simulink model "state_obsv"  (R2020b)
settings: Solver=VariableStepAuto  StartTime=0.0  StopTime=1  MaxStep=1e-3  RelTol=1e-3
values from neighbouring files (symbols this model uses):
  A = [-R/L -1/L; 1/Ca 0]    [E1_1.m]    (also in E3_5.m = [-299 37;-2416 299]; E5_1.m = [0 0 1; 2 -1 2; 0 1 1]; E_140421_1.m = [0 -1; 3 -2]; E_140421_2.m = [3 2; 0 -5])
  alpha = 1    [Reg.m]    (also in State_feed.m = [-(C-D*K)*(A-B*K)^-1*B+D]^-1)
  B = [1/L 0]'    [E1_1.m]    (also in E3_5.m = [7 57]'; E_140421_1.m = [1 1]'; E_140421_2.m = [1 0]'; E_280421_1.m = [1;2])
  C = [0 1]    [E1_1.m]    (also in E5_1.m = [0 0 1]; E_140421_1.m = [1 1]; E_140421_2.m = [1 1]; E_280421_1.m = [1 -1])
  K = place(A,B,[-1 -7])    [E3_5.m]    (also in E_140421_1.m = place(A,B,[20 -10]); Esempi.m = place(A,B,[-1,-2,-3]); EserciziFinali.m = place(A,B,[20, -10]); Problem_P2.m = 20*log10(m))
  L = 2e-3    (= 0.002)    [E1_1.m]    (also in E5_1.m = Lt'; Esempi.m = place(A',C',[0.05 0.1 0.2])'; EserciziFinali.m = place(A',C',[-10 -20])'; Exam_202007.m = Gc*Gp*Gs*Ga*Gf)
libraries: simulink x1
settings Model: Creator=kevin  LastModifiedBy=kevin

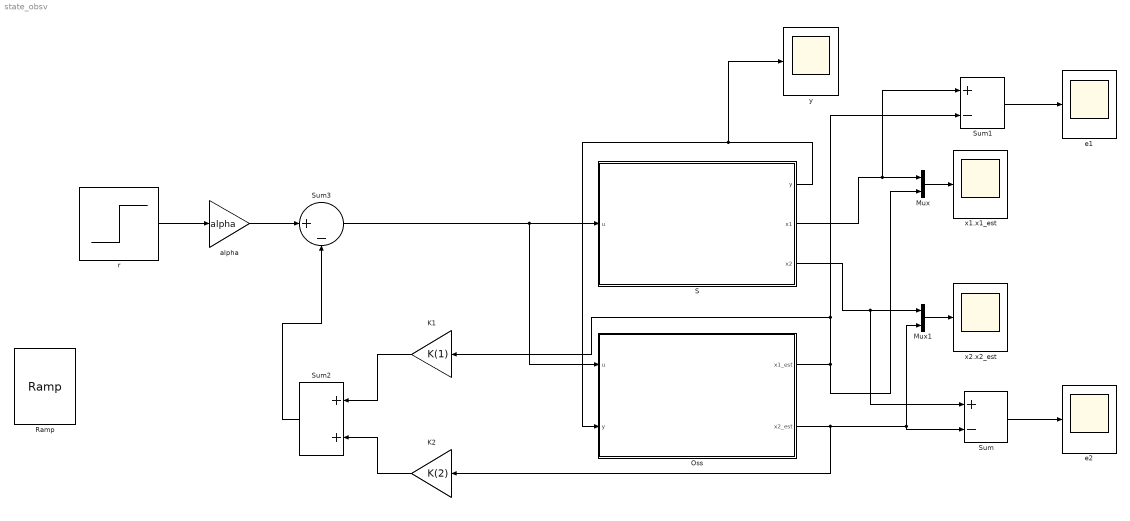
== system state_obsv ==
  K1 : Gain  Gain=K(1)
  K2 : Gain  Gain=K(2)
  Mux : Mux  Inputs=2
  Mux1 : Mux  Inputs=2
  Oss : Subsystem
  Ramp : simulink/Sources/Ramp  slope=1  start=0  InitialOutput=0
  S : Subsystem
  Sum : Sum  Inputs=+-
  Sum1 : Sum  Inputs=+-
  Sum2 : Sum
  Sum3 : Sum  Inputs=|+-
  alpha : Gain  Gain=alpha
  e1 : Scope
  e2 : Scope
  r : Step  Time=0  SampleTime=0
  x1.x1_est : Scope
  x2.x2_est : Scope
  y : Scope
  wires:
  Mux/1 -> x1.x1_est/1
  Mux1/1 -> x2.x2_est/1
  S/2(x1) -> Sum1/1, Mux/1
  S/3(x2) -> Sum/1, Mux1/1
  Oss/2(x2_est) -> K2/1, Sum/2, Mux1/2
  S/1(y) -> y/1, Oss/2(y)
  Sum1/1 -> e1/1
  Sum/1 -> e2/1
  Oss/1(x1_est) -> Mux/2, K1/1, Sum1/2
  r/1 -> alpha/1
  alpha/1 -> Sum3/1
  Sum2/1 -> Sum3/2
  K2/1 -> Sum2/2
  K1/1 -> Sum2/1
  Sum3/1 -> Oss/1(u), S/1(u)

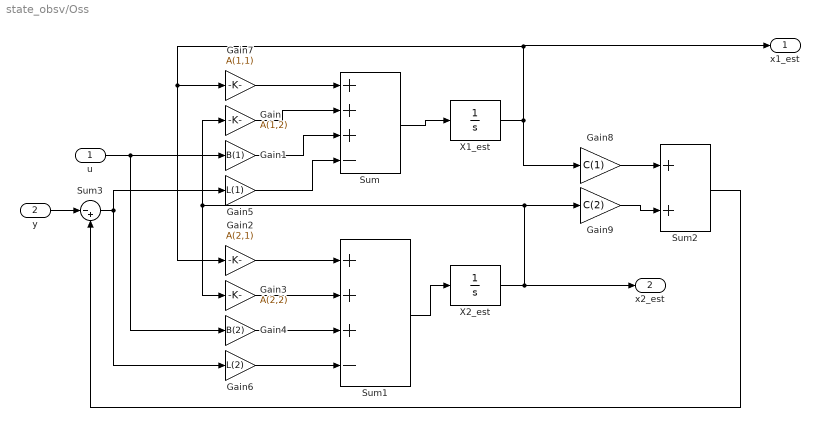
== system state_obsv/Oss ==
  u : Inport
  y : Inport  Port=2
  Gain : Gain  Gain=A(1,2)
  Gain1 : Gain  Gain=B(1)
  Gain2 : Gain  Gain=A(2,1)
  Gain3 : Gain  Gain=A(2,2)
  Gain4 : Gain  Gain=B(2)
  Gain5 : Gain  Gain=L(1)
  Gain6 : Gain  Gain=L(2)
  Gain7 : Gain  Gain=A(1,1)
  Gain8 : Gain  Gain=C(1)
  Gain9 : Gain  Gain=C(2)
  Sum : Sum  Inputs=+++-
  Sum1 : Sum  Inputs=+++-
  Sum2 : Sum
  Sum3 : Sum  Inputs=|-+
  X1_est : Integrator
  X2_est : Integrator
  x1_est : Outport
  x2_est : Outport  Port=2
  wires:
  Gain4/1 -> Sum1/3
  Sum/1 -> X1_est/1
  X2_est/1 -> x2_est/1, Gain9/1, Gain3/1, Gain/1
  Gain3/1 -> Sum1/2
  Sum1/1 -> X2_est/1
  Gain/1 -> Sum/2
  Gain1/1 -> Sum/3
  u/1 -> Gain4/1, Gain1/1
  X1_est/1 -> Gain8/1, Gain7/1, Gain2/1, x1_est/1
  Gain2/1 -> Sum1/1
  Sum2/1 -> Sum3/2
  y/1 -> Sum3/1
  Sum3/1 -> Gain6/1, Gain5/1
  Gain5/1 -> Sum/4
  Gain6/1 -> Sum1/4
  Gain7/1 -> Sum/1
  Gain8/1 -> Sum2/1
  Gain9/1 -> Sum2/2

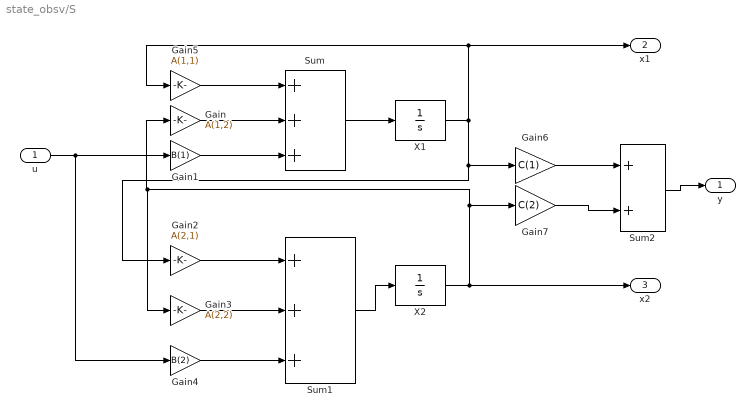
== system state_obsv/S ==
  u : Inport
  Gain : Gain  Gain=A(1,2)
  Gain1 : Gain  Gain=B(1)
  Gain2 : Gain  Gain=A(2,1)
  Gain3 : Gain  Gain=A(2,2)
  Gain4 : Gain  Gain=B(2)
  Gain5 : Gain  Gain=A(1,1)
  Gain6 : Gain  Gain=C(1)
  Gain7 : Gain  Gain=C(2)
  Sum : Sum  Inputs=+++
  Sum1 : Sum  Inputs=+++
  Sum2 : Sum
  X1 : Integrator  InitialCondition=-5
  X2 : Integrator  InitialCondition=1
  y : Outport
  x1 : Outport  Port=2
  x2 : Outport  Port=3
  wires:
  Gain4/1 -> Sum1/3
  Sum/1 -> X1/1
  X2/1 -> x2/1, Gain7/1, Gain3/1, Gain/1
  Gain3/1 -> Sum1/2
  Sum1/1 -> X2/1
  Gain/1 -> Sum/2
  Gain1/1 -> Sum/3
  u/1 -> Gain4/1, Gain1/1
  X1/1 -> Gain5/1, x1/1, Gain6/1, Gain2/1
  Gain2/1 -> Sum1/1
  Sum2/1 -> y/1
  Gain5/1 -> Sum/1
  Gain6/1 -> Sum2/1
  Gain7/1 -> Sum2/2
